simulink model "R_soft_sim"  (R2021a)
settings: Solver=ode5  StartTime=0.0  StopTime=30.0  FixedStep=0.000001  RelTol=1e-3
values from neighbouring files (symbols this model uses):
  beta = 0.1    [computational_time.m]    (also in final_simulation.m; init_script.m)
  beta_r = 0.5    [final_simulation.m]
  D = 0.1    [computational_time.m]    (also in dampingMatrix.m = reshape([0.0,0.0,0.0,0.0,beta,t2,0.0,t2,beta./3.0],[3,3]); final_simulation.m; init_script.m; multiple_frame_plot.m)
  g = 9.81    [computational_time.m]    (also in final_simulation.m; init_script.m)
  k = 1    [computational_time.m]    (also in final_simulation.m; init_script.m = 0.1)
  L = 1    [computational_time.m]    (also in coriolisMatrix.m = ct{1}; final_simulation.m; init_script.m; multiple_frame_plot.m)
  m = 1    [computational_time.m]    (also in coriolisMatrix.m = ct{2}; final_simulation.m; init_script.m)
  theta_dot_init = zeros(3, 1)    [final_simulation.m]
  theta_init = [0; pi/4; -pi/4]    [final_simulation.m]
undefined symbols (not defined in the file or in its folder): RSoft_dynamics, Soft_dynamics
settings Model: Creator=Utente  LastModifiedBy=Utente

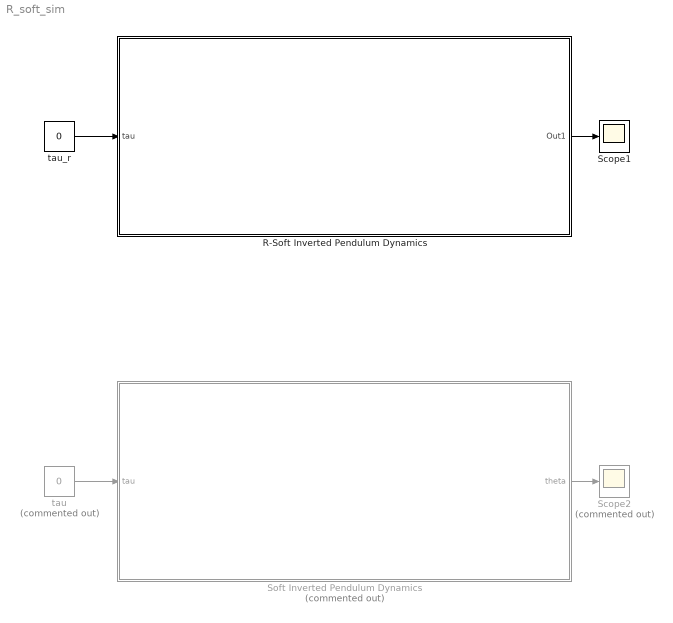
== system R_soft_sim ==
  R-Soft Inverted Pendulum Dynamics : Subsystem
  Scope1 : Scope
  Scope2 : Scope  Commented=on
  Soft Inverted Pendulum Dynamics : Subsystem  Commented=on
  tau : Constant  Commented=on  Value=0
  tau_r : Constant  Value=0
  wires:
  tau/1 -> Soft Inverted Pendulum Dynamics/1(tau)
  Soft Inverted Pendulum Dynamics/1(theta) -> Scope2/1
  tau_r/1 -> R-Soft Inverted Pendulum Dynamics/1(tau)
  R-Soft Inverted Pendulum Dynamics/1(Out1) -> Scope1/1

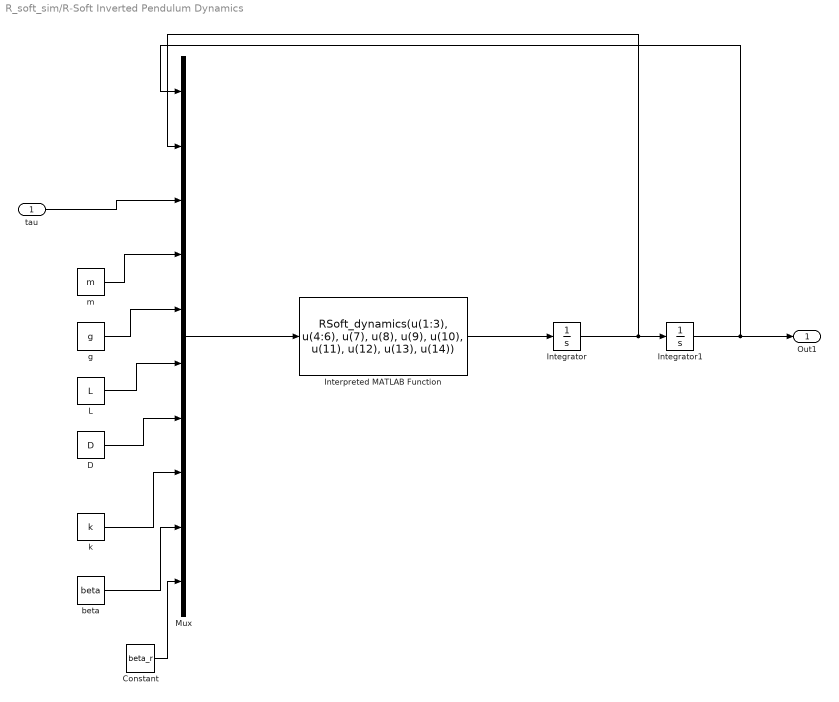
== system R_soft_sim/R-Soft Inverted Pendulum Dynamics ==
  tau : Inport
  Constant : Constant  Value=beta_r
  D : Constant  Value=D
  Integrator : Integrator  InitialCondition=theta_dot_init
  Integrator1 : Integrator  InitialCondition=theta_init
  Interpreted MATLAB Function : MATLABFcn  MATLABFcn=RSoft_dynamics(u(1:3), u(4:6), u(7), u(8), u(9), u(10), u(11), u(12), u(13), u(14))
  L : Constant  Value=L
  Mux : Mux  Inputs=10
  beta : Constant  Value=beta
  g : Constant  Value=g
  k : Constant  Value=k
  m : Constant  Value=m
  Out1 : Outport
  wires:
  Integrator1/1 -> Out1/1, Mux/1
  g/1 -> Mux/5
  beta/1 -> Mux/9
  k/1 -> Mux/8
  m/1 -> Mux/4
  tau/1 -> Mux/3
  Integrator/1 -> Mux/2, Integrator1/1
  L/1 -> Mux/6
  D/1 -> Mux/7
  Mux/1 -> Interpreted MATLAB Function/1
  Interpreted MATLAB Function/1 -> Integrator/1
  Constant/1 -> Mux/10

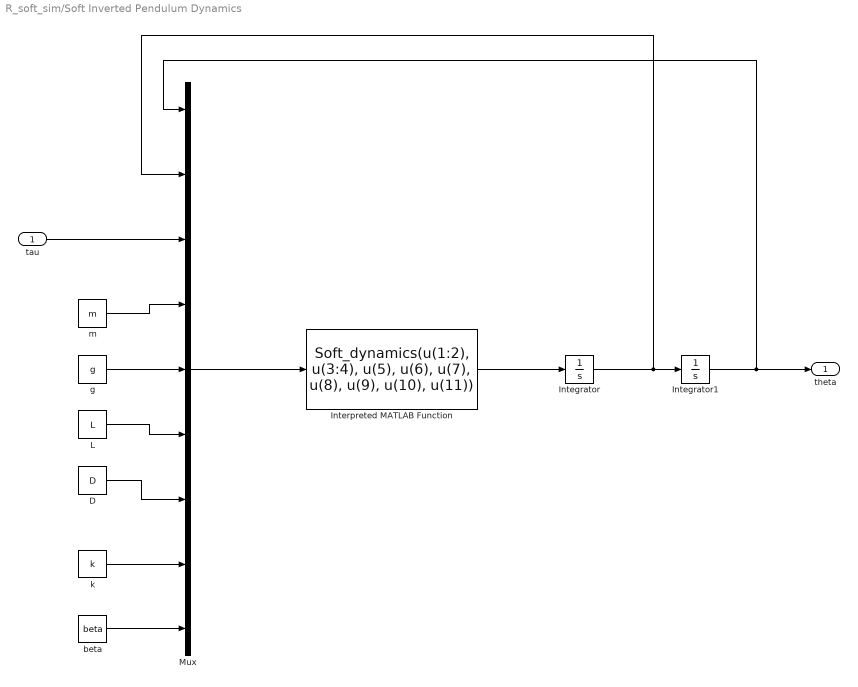
== system R_soft_sim/Soft Inverted Pendulum Dynamics ==
  tau : Inport
  D : Constant  Value=D
  Integrator : Integrator  InitialCondition=[0; 0]
  Integrator1 : Integrator  InitialCondition=[pi/4; -pi/4]
  Interpreted MATLAB Function : MATLABFcn  MATLABFcn=Soft_dynamics(u(1:2), u(3:4), u(5), u(6), u(7), u(8), u(9), u(10), u(11))
  L : Constant  Value=L
  Mux : Mux  Inputs=9
  beta : Constant  Value=beta
  g : Constant  Value=g
  k : Constant  Value=k
  m : Constant  Value=m
  theta : Outport
  wires:
  Integrator1/1 -> theta/1, Mux/1
  g/1 -> Mux/5
  beta/1 -> Mux/9
  k/1 -> Mux/8
  m/1 -> Mux/4
  tau/1 -> Mux/3
  Integrator/1 -> Mux/2, Integrator1/1
  L/1 -> Mux/6
  D/1 -> Mux/7
  Mux/1 -> Interpreted MATLAB Function/1
  Interpreted MATLAB Function/1 -> Integrator/1
